simulink model "SimulinkOminidirectinalDrone"  (R2025a)
settings: Solver=ode15s  StartTime=0.0  StopTime=10  RelTol=1e-4
values from neighbouring files (symbols this model uses):
  AUM = 3.057    [Parameter.m]
  Cq = 0.013    [Parameter.m]
  Ct = 0.013    [Parameter.m]
  g = 10    [Parameter.m]
  H = 0.05    [Parameter.m]
  Ixx = 0.049827    [Parameter.m]
  Iyy = 0.048993    [Parameter.m]
  Izz = 0.082777    [Parameter.m]
  L = 0.3    [Parameter.m]
  rho = 1.18195    [Parameter.m]
  W = diag([0.994, 0.003, 0.003, 0.994, 0.003, 0.003,            0.994, 0.003, 0.003, 0.994, 0.003, 0.003])    [Parameter.m]
undefined symbols (not defined in the file or in its folder): R_rad
libraries: sharedutil x4, aerolibobsolete x1
(part 2 of 2)

== matlab function SimulinkOminidirectinalDrone/Vehicle Dynamic/actuator/Arm2/STANDARD ARM MODEL CLOCKWISE/MATLAB Function1 ==
  data: eta input; M output; etadot input; etadotdot input; gamma input; gammadot input; gammadotdot input; omega input; omegadot input; p input; q input; r input; pdot input; qdot input; rdot input; Ixx input; Iyy input; Izz input
function M = fcn(eta,etadot,etadotdot,gamma,gammadot,gammadotdot,omega,omegadot, p,q,r,pdot,qdot,rdot,Ixx,Iyy,Izz)

M1reactX = (1/4)*(-2*Ixx*q*r+Iyy*q*r+Izz*q*r+3*Iyy*cos(2*gamma)*q*r-3*cos(2*gamma)*q*r-...
    4*Izz*sin(gamma)*omega*r+2*Iyy*etadot*r+2*Izz*etadot+2*Iyy*cos(2*gamma)*etadot*r-2*Izz*cos(2*gamma)*etadot*r-2*Ixx*pdot-Iyy*pdot...
    -Izz*pdot+Iyy*cos(2*gamma)*pdot-Izz*cos(2*gamma)*pdot-2*Iyy*p*sin(2*gamma)*gammadot+2*Izz*p*sin(2*gamma)*gammadot...
    -sin(2*eta)*(4*(Ixx-Iyy)*p*sin(gamma)*omega+2*(Iyy-Izz)*r*sin(2*gamma)*gammadot-(2*Ixx-Iyy-Izz)*(rdot+p*(q+2*etadot))...
    -(Iyy-Izz)*cos(2*eta)*(rdot+p*(q+2*etadot)))-cos(2*eta)*(4*(Ixx-Iyy)*r*sin(gamma)*omega+2*(Izz-Iyy)*p*sin(2*gamma)*gammadot...
    +(2*Ixx-Iyy-Izz)*(pdot-r*(q+2*etadot))+(Iyy-Izz)*cos(2*gamma)*(pdot-r*(q+2*etadot)))...
    -2*cos(eta)*(2*(Ixx-Iyy+Izz)*cos(gamma)*omega*(q+etadot)+(Iyy-Izz)*sin(2*gamma)*(q-r+etadot)*...
    (q+r+etadot)+2*Ixx*gammadotdot)-2*sin(eta)*(-2*(-Ixx+Iyy+Izz)*sin(gamma)*omega*gammadot-2*Ixx*(q+etadot)*gammadot+2*(Iyy-Izz)*...
    cos(2*gamma)*(q+etadot)*gammadot+2*Izz*cos(gamma)*omegadot-(Iyy-Izz)*sin(2*gamma)*(p*r-qdot-etadotdot)));

M1reactY = (1/4)*(-2*Ixx*sin(2*eta)*p^2+Iyy*sin(2*eta)*p^2+Izz*sin(2*eta)*p^2-4*Ixx*cos(2*eta)*r*p+...
    2*Iyy*cos(2*eta)*r*p+2*Izz*cos(2*eta)*r*p-4*Ixx*sin(eta)*gammadot*p+2*Ixx*r^2*sin(2*eta)-...
    Iyy*r^2*sin(2*eta)-Izz*r^2*sin(2*eta)-2*Iyy*qdot-2*Izz*qdot-4*Ixx*cos(eta)*r*gammadot-4*(Ixx-Iyy-Izz)*cos(gamma)*omega*(cos(eta)*p...
    -r*sin(eta)+gammadot)+2*(Iyy-Izz)*sin(2*gamma)*(-sin(eta)*(q*r+pdot)+cos(eta)*(p*q-rdot)+2*gammadot*(q+etadot))+4*Izz*sin(gamma)*...
    omegadot-2*Iyy*etadotdot-2*Izz*etadotdot-2*(Iyy-Izz)*cos(2*gamma)*(qdot+(cos(eta)*r+p*sin(eta))*(cos(eta)*p-r*sin(eta)+2*gammadot)+etadotdot));

M1reactZ = (1/4)*(-2*(Iyy-Izz)*sin(2*gamma)*sin(eta)*p^2-(4*(Iyy-Izz)*cos(2*gamma)*etadot*(sin(eta)^2+...
    (2*(-2*Ixx+Iyy+Izz)*(cos(eta)^2)-(Iyy-Izz)*cos(2*gamma)*(cos(2*eta)-3))*q...
    -4*(Izz+(Iyy-Ixx)*cos(2*eta))*sin(gamma)*omega+2*(Iyy-Izz)*cos(eta)*sin(2*gamma)*(r+2*sin(eta)*gammadot)+...
    2*(Iyy+Izz+(-2*Ixx+Iyy+Izz)*cos(2*eta))*etadot)*p-2*Ixx*rdot-Iyy*rdot-Izz*rdot+Iyy*cos(2*gamma)*...
    rdot-Izz*cos(2*gamma)*rdot-2*Iyy*r*sin(2*gamma)*gammadot+2*Izz*r*sin(2*gamma)*gammadot-cos(2*gamma)*((-2*Ixx+Iyy+Izz+(Izz-Iyy)*cos(2*gamma))*rdot+...
    2*(Iyy-Izz)*r*sin(2*gamma)*gammadot)-sin(2*eta)*(4*(Iyy-Ixx)*r*sin(gamma)*omega+(2*Ixx-Iyy-Izz)*(r*(q+2*etadot)-pdot)...
    +(Iyy-Izz)*cos(2*gamma)*(r*(q+2*etadot)-pdot))-2*sin(eta)*(-(Iyy-Izz)*sin(2*gamma)*(q+etadot)^2 ...
    -2*(Ixx-Iyy+Izz)*cos(gamma)*omega*(q+etadot)-2*Ixx*gammadotdot)-2*cos(eta)*(-2*(-Ixx+Iyy+Izz)*sin(gamma)*omega*gammadot...
    -2*Ixx*(q+etadot)*gammadot)+2*(Iyy-Izz)*cos(2*gamma)*(q+etadot)*gammadot+2*Izz*cos(gamma)*omegadot+(Iyy-Izz)*sin(2*gamma)*(qdot+etadotdot)));

M = [ M1reactX;
      M1reactY;
      M1reactZ];

== matlab function SimulinkOminidirectinalDrone/Vehicle Dynamic/actuator/Arm 3/STANDARD ARM MODEL CLOCKWISE/MATLAB Function1 ==
  data: eta input; M output; etadot input; etadotdot input; gamma input; gammadot input; gammadotdot input; omega input; omegadot input; p input; q input; r input; pdot input; qdot input; rdot input; Ixx input; Iyy input; Izz input
function M = fcn(eta,etadot,etadotdot,gamma,gammadot,gammadotdot,omega,omegadot, p,q,r,pdot,qdot,rdot,Ixx,Iyy,Izz)

M1reactX = (1/4)*(-2*Ixx*q*r+Iyy*q*r+Izz*q*r+3*Iyy*cos(2*gamma)*q*r-3*cos(2*gamma)*q*r-...
    4*Izz*sin(gamma)*omega*r+2*Iyy*etadot*r+2*Izz*etadot+2*Iyy*cos(2*gamma)*etadot*r-2*Izz*cos(2*gamma)*etadot*r-2*Ixx*pdot-Iyy*pdot...
    -Izz*pdot+Iyy*cos(2*gamma)*pdot-Izz*cos(2*gamma)*pdot-2*Iyy*p*sin(2*gamma)*gammadot+2*Izz*p*sin(2*gamma)*gammadot...
    -sin(2*eta)*(4*(Ixx-Iyy)*p*sin(gamma)*omega+2*(Iyy-Izz)*r*sin(2*gamma)*gammadot-(2*Ixx-Iyy-Izz)*(rdot+p*(q+2*etadot))...
    -(Iyy-Izz)*cos(2*eta)*(rdot+p*(q+2*etadot)))-cos(2*eta)*(4*(Ixx-Iyy)*r*sin(gamma)*omega+2*(Izz-Iyy)*p*sin(2*gamma)*gammadot...
    +(2*Ixx-Iyy-Izz)*(pdot-r*(q+2*etadot))+(Iyy-Izz)*cos(2*gamma)*(pdot-r*(q+2*etadot)))...
    -2*cos(eta)*(2*(Ixx-Iyy+Izz)*cos(gamma)*omega*(q+etadot)+(Iyy-Izz)*sin(2*gamma)*(q-r+etadot)*...
    (q+r+etadot)+2*Ixx*gammadotdot)-2*sin(eta)*(-2*(-Ixx+Iyy+Izz)*sin(gamma)*omega*gammadot-2*Ixx*(q+etadot)*gammadot+2*(Iyy-Izz)*...
    cos(2*gamma)*(q+etadot)*gammadot+2*Izz*cos(gamma)*omegadot-(Iyy-Izz)*sin(2*gamma)*(p*r-qdot-etadotdot)));

M1reactY = (1/4)*(-2*Ixx*sin(2*eta)*p^2+Iyy*sin(2*eta)*p^2+Izz*sin(2*eta)*p^2-4*Ixx*cos(2*eta)*r*p+...
    2*Iyy*cos(2*eta)*r*p+2*Izz*cos(2*eta)*r*p-4*Ixx*sin(eta)*gammadot*p+2*Ixx*r^2*sin(2*eta)-...
    Iyy*r^2*sin(2*eta)-Izz*r^2*sin(2*eta)-2*Iyy*qdot-2*Izz*qdot-4*Ixx*cos(eta)*r*gammadot-4*(Ixx-Iyy-Izz)*cos(gamma)*omega*(cos(eta)*p...
    -r*sin(eta)+gammadot)+2*(Iyy-Izz)*sin(2*gamma)*(-sin(eta)*(q*r+pdot)+cos(eta)*(p*q-rdot)+2*gammadot*(q+etadot))+4*Izz*sin(gamma)*...
    omegadot-2*Iyy*etadotdot-2*Izz*etadotdot-2*(Iyy-Izz)*cos(2*gamma)*(qdot+(cos(eta)*r+p*sin(eta))*(cos(eta)*p-r*sin(eta)+2*gammadot)+etadotdot));

M1reactZ = (1/4)*(-2*(Iyy-Izz)*sin(2*gamma)*sin(eta)*p^2-(4*(Iyy-Izz)*cos(2*gamma)*etadot*(sin(eta)^2+...
    (2*(-2*Ixx+Iyy+Izz)*(cos(eta)^2)-(Iyy-Izz)*cos(2*gamma)*(cos(2*eta)-3))*q...
    -4*(Izz+(Iyy-Ixx)*cos(2*eta))*sin(gamma)*omega+2*(Iyy-Izz)*cos(eta)*sin(2*gamma)*(r+2*sin(eta)*gammadot)+...
    2*(Iyy+Izz+(-2*Ixx+Iyy+Izz)*cos(2*eta))*etadot)*p-2*Ixx*rdot-Iyy*rdot-Izz*rdot+Iyy*cos(2*gamma)*...
    rdot-Izz*cos(2*gamma)*rdot-2*Iyy*r*sin(2*gamma)*gammadot+2*Izz*r*sin(2*gamma)*gammadot-cos(2*gamma)*((-2*Ixx+Iyy+Izz+(Izz-Iyy)*cos(2*gamma))*rdot+...
    2*(Iyy-Izz)*r*sin(2*gamma)*gammadot)-sin(2*eta)*(4*(Iyy-Ixx)*r*sin(gamma)*omega+(2*Ixx-Iyy-Izz)*(r*(q+2*etadot)-pdot)...
    +(Iyy-Izz)*cos(2*gamma)*(r*(q+2*etadot)-pdot))-2*sin(eta)*(-(Iyy-Izz)*sin(2*gamma)*(q+etadot)^2 ...
    -2*(Ixx-Iyy+Izz)*cos(gamma)*omega*(q+etadot)-2*Ixx*gammadotdot)-2*cos(eta)*(-2*(-Ixx+Iyy+Izz)*sin(gamma)*omega*gammadot...
    -2*Ixx*(q+etadot)*gammadot)+2*(Iyy-Izz)*cos(2*gamma)*(q+etadot)*gammadot+2*Izz*cos(gamma)*omegadot+(Iyy-Izz)*sin(2*gamma)*(qdot+etadotdot)));

M = [ M1reactX;
      M1reactY;
      M1reactZ];

== matlab function SimulinkOminidirectinalDrone/Vehicle Dynamic/actuator/Arm 3/STANDARD ARM MODEL CLOCKWISE/prop behaviour ==
  data: Omega input; Ct input; Cq input; rho input; F output; R input; M output
function [F, M] = fcn(Omega, Ct, Cq, rho, R)
%#codegen
% Inputs:
%   rho   - air density (kg/m^3)
%   R     - propeller radius (m)
%   Omega - angular velocity (rad/s)
%   Ct    - thrust coefficient
%   Cq    - torque coefficient
%
% Outputs:
%   T - Thrust force (N)
%   Q - Torque (Nm)
% Rotor disk area
A = pi * R^2;
% Thrust (eq. 4.38)
F = [0; 0; rho * A * (Omega * R)^2 * Ct];
% Torque (eq. 4.39)
M = [0; 0; rho * A * (Omega * R)^2 * R * Cq];

end
